simulink model "ProposedProblem1"  (R2013a)
settings: Solver=ode45  StartTime=0.0  StopTime=50  RelTol=1e-3
undefined symbols (not defined in the file): des, gcbh
settings Model: Creator=gabig  LastModifiedBy=gabig

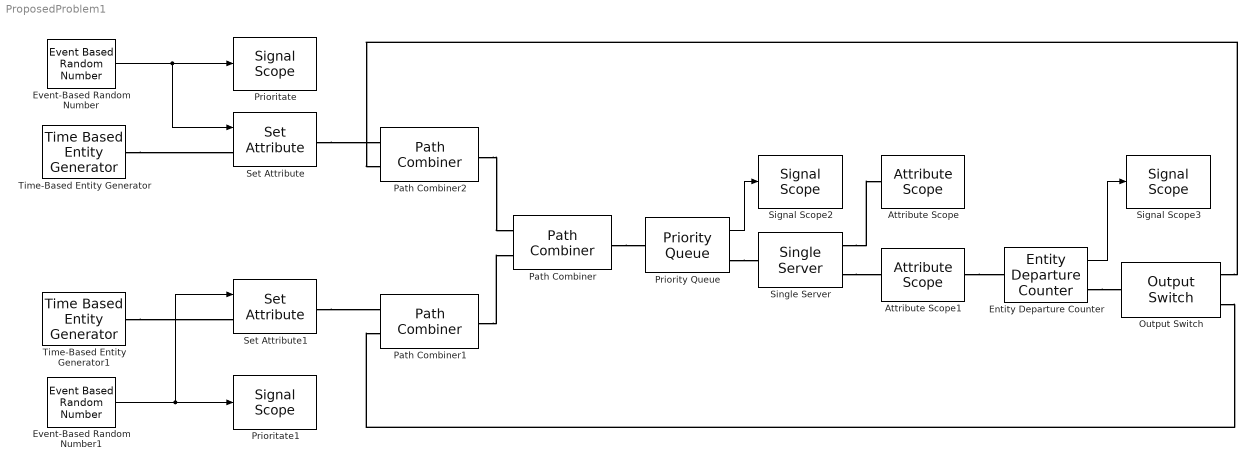
== system ProposedProblem1 ==
  Attribute Scope : AttributeScope  LoadFcn=des.scope.CallbackSupport('seLoadFcn',gcbh)  StartFcn=des.scope.CallbackSupport('seStartFcn',gcbh)  StopFcn=des.scope.CallbackSupport('seStopFcn',gcbh)
      settings: CopyFcn=des.scope.CallbackSupport('seCopyFcn',gcbh)  DeleteFcn=des.scope.CallbackSupport('seDeleteFcn',gcbh)  PreSaveFcn=des.scope.CallbackSupport('sePreSaveFcn',gcbh)  NameChangeFcn=des.scope.CallbackSupport('seNameChangeFcn',gcbh)  OpenFcn=des.scope.CallbackSupport('seOpenFcn',gcbh)
  Attribute Scope1 : AttributeScope  LoadFcn=des.scope.CallbackSupport('seLoadFcn',gcbh)  StartFcn=des.scope.CallbackSupport('seStartFcn',gcbh)  StopFcn=des.scope.CallbackSupport('seStopFcn',gcbh)
      settings: CopyFcn=des.scope.CallbackSupport('seCopyFcn',gcbh)  DeleteFcn=des.scope.CallbackSupport('seDeleteFcn',gcbh)  PreSaveFcn=des.scope.CallbackSupport('sePreSaveFcn',gcbh)  NameChangeFcn=des.scope.CallbackSupport('seNameChangeFcn',gcbh)  OpenFcn=des.scope.CallbackSupport('seOpenFcn',gcbh)
  Entity Departure Counter : EntityDepartureCounter  NumberDepartedToSignal=on
  Event-Based Random Number : EventBasedRandomNumber  Seed=12344
  Event-Based Random Number1 : EventBasedRandomNumber  Seed=12448
  Output Switch : OutputSwitch  NumberOutputPorts=2  SwitchingCriterion=From attribute  AttributeName=Tip_task
  Path Combiner : PathCombiner  NumberInputPorts=2
  Path Combiner1 : PathCombiner  NumberInputPorts=2
  Path Combiner2 : PathCombiner  NumberInputPorts=2
  Prioritate : SignalScope  LoadFcn=des.scope.CallbackSupport('seLoadFcn',gcbh)  StartFcn=des.scope.CallbackSupport('seStartFcn',gcbh)  StopFcn=des.scope.CallbackSupport('seStopFcn',gcbh)
      settings: CopyFcn=des.scope.CallbackSupport('seCopyFcn',gcbh)  DeleteFcn=des.scope.CallbackSupport('seDeleteFcn',gcbh)  PreSaveFcn=des.scope.CallbackSupport('sePreSaveFcn',gcbh)  NameChangeFcn=des.scope.CallbackSupport('seNameChangeFcn',gcbh)  OpenFcn=des.scope.CallbackSupport('seOpenFcn',gcbh)
  Prioritate1 : SignalScope  LoadFcn=des.scope.CallbackSupport('seLoadFcn',gcbh)  StartFcn=des.scope.CallbackSupport('seStartFcn',gcbh)  StopFcn=des.scope.CallbackSupport('seStopFcn',gcbh)
      settings: CopyFcn=des.scope.CallbackSupport('seCopyFcn',gcbh)  DeleteFcn=des.scope.CallbackSupport('seDeleteFcn',gcbh)  PreSaveFcn=des.scope.CallbackSupport('sePreSaveFcn',gcbh)  NameChangeFcn=des.scope.CallbackSupport('seNameChangeFcn',gcbh)  OpenFcn=des.scope.CallbackSupport('seOpenFcn',gcbh)
  Priority Queue : PriorityQueue  SortingAttributeName=Prioritate  StatAverageQueueLength=on
      settings: OutputPortMap=o3
  Set Attribute : SetAttribute  AttributeName=Prioritate|Timp_deservire|Tip_task  AttributeFrom=Signal port|Dialog|Dialog  AttributeValue=1|1|1  AttributeTreatAsVector=1|1|1  EvaluatedAttributeValue={ [];1;1}
  Set Attribute1 : SetAttribute  AttributeName=Prioritate|Timp_deservire|Tip_task  AttributeFrom=Signal port|Dialog|Dialog  AttributeValue=1|2.5|2  AttributeTreatAsVector=1|1|1  EvaluatedAttributeValue={ [];2.5;2}
  Signal Scope2 : SignalScope  LoadFcn=des.scope.CallbackSupport('seLoadFcn',gcbh)  StartFcn=des.scope.CallbackSupport('seStartFcn',gcbh)  StopFcn=des.scope.CallbackSupport('seStopFcn',gcbh)
      settings: CopyFcn=des.scope.CallbackSupport('seCopyFcn',gcbh)  DeleteFcn=des.scope.CallbackSupport('seDeleteFcn',gcbh)  PreSaveFcn=des.scope.CallbackSupport('sePreSaveFcn',gcbh)  NameChangeFcn=des.scope.CallbackSupport('seNameChangeFcn',gcbh)  OpenFcn=des.scope.CallbackSupport('seOpenFcn',gcbh)
  Signal Scope3 : SignalScope  LoadFcn=des.scope.CallbackSupport('seLoadFcn',gcbh)  StartFcn=des.scope.CallbackSupport('seStartFcn',gcbh)  StopFcn=des.scope.CallbackSupport('seStopFcn',gcbh)
      settings: CopyFcn=des.scope.CallbackSupport('seCopyFcn',gcbh)  DeleteFcn=des.scope.CallbackSupport('seDeleteFcn',gcbh)  PreSaveFcn=des.scope.CallbackSupport('sePreSaveFcn',gcbh)  NameChangeFcn=des.scope.CallbackSupport('seNameChangeFcn',gcbh)  OpenFcn=des.scope.CallbackSupport('seOpenFcn',gcbh)
  Single Server : SingleServer  ServiceTimeFrom=Attribute  AttributeName=Timp_deservire  PermitPreemption=on  SortingAttributeName=Prioritate  WriteToAttribute=on
  Time-Based Entity Generator : TimeBasedEntityGenerator  Period=2
  Time-Based Entity Generator1 : TimeBasedEntityGenerator  Period=5
  wires:
  Event-Based Random Number/1 -> Set Attribute/1, Prioritate/1
  Event-Based Random Number1/1 -> Set Attribute1/1, Prioritate1/1
  Entity Departure Counter/1 -> Signal Scope3/1
  Priority Queue/1 -> Signal Scope2/1
  connections:
  Single Server/RConn2 -- Attribute Scope1/LConn1
  Set Attribute/RConn1 -- Path Combiner2/LConn1
  Path Combiner2/RConn1 -- Path Combiner/LConn1
  Set Attribute1/RConn1 -- Path Combiner1/LConn1
  Attribute Scope1/RConn1 -- Entity Departure Counter/LConn1
  Priority Queue/RConn1 -- Single Server/LConn1
  Path Combiner1/RConn1 -- Path Combiner/LConn2
  Time-Based Entity Generator1/RConn1 -- Set Attribute1/LConn1
  Single Server/RConn1 -- Attribute Scope/LConn1
  Output Switch/RConn2 -- Path Combiner1/LConn2
  Time-Based Entity Generator/RConn1 -- Set Attribute/LConn1
  Output Switch/RConn1 -- Path Combiner2/LConn2
  Entity Departure Counter/RConn1 -- Output Switch/LConn1
  Path Combiner/RConn1 -- Priority Queue/LConn1
